simulink model "PIL_System_POTS"  (R2025b)
settings: Solver=FixedStepAuto  StartTime=0.0  StopTime=10.0  RelTol=1e-3  EnableMultiTasking=on
libraries: stm32f4xxblockslib x2
settings Model: STM32="{\"AnalogInput\":[{\"ID\":\"PIL_System_POTS:37\"},{\"ID\":\"PIL_System_POTS:38\"}]}"  Creator=Lakshay Taneja  LastModifiedBy=Lakshay Taneja
settings OptimizationCC: DefaultParameterBehavior=Inlined  EnhancedBackFolding=on  PassReuseOutputArgsAs=Individual arguments  ZeroExternalMemoryAtStartup=off  ZeroInternalMemoryAtStartup=off  MaxStackSize=512  OptimizeBlockOrder=speed  DifferentSizesBufferReuse=on  OptimizationCustomize=off  EfficientTunableParamExpr=on
settings DebuggingCC: ParameterTunabilityLossMsg=error
settings HardwareCC: ProdBitPerPointer=32.0  ProdBitPerSizeT=32.0  ProdBitPerPtrDiffT=32.0  ProdLargestAtomicInteger=Long  ProdLargestAtomicFloat=Double  ProdWordSize=32.0  ProdLongLongMode=on  ProdHWDeviceType=ARM Compatible->ARM Cortex-M
settings SFSimCC: MATLABDynamicMemAlloc=off
settings RTWCC: SystemTargetFile=ert.tlc  HardwareBoard=STM32F4xx Based  TemplateMakefile=ert_default_tmf  Toolchain=GNU Tools for ARM Embedded Processors  CreateSILPILBlock=PIL  Description=Embedded Coder
settings CodeAppCC: ForceParamTrailComments=on  IgnoreCustomStorageClasses=off  OperatorAnnotations=on  SimulinkDataObjDesc=on  SFDataObjDesc=on  InsertBlockDesc=on
settings ERTTargetCC: ExtModeTransport=3.0  ExtModeStaticAlloc=on  ExtModeStaticAllocSize=2048.0  ExtModeMexFile=ext_xcp  ExtModeIntrfLevel=Level2 - Open  TargetLangStandard=C99 (ISO)  CodeReplacementLibrary=ARM Cortex-M

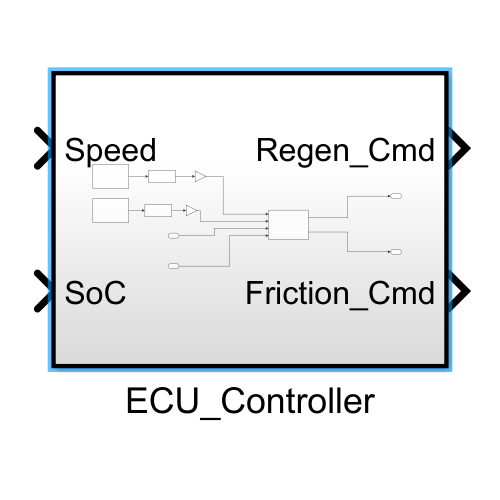
[thumbnail: Simulink's stored preview of the top-level diagram]
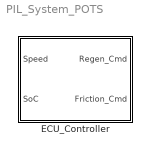
== system PIL_System_POTS ==
  ECU_Controller : Subsystem  TreatAsAtomicUnit=on

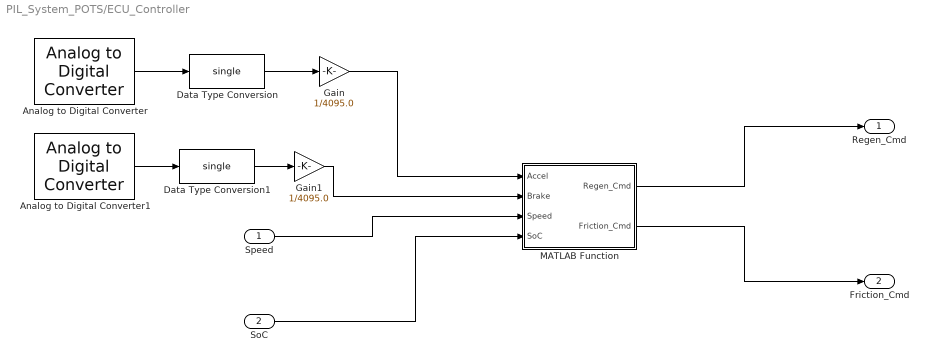
== system PIL_System_POTS/ECU_Controller ==
  Speed : Inport  OutDataTypeStr=single
  SoC : Inport  Port=2  OutDataTypeStr=single
  Analog to Digital Converter : stm32f4xxblockslib/Analog to Digital Converter  ADCModule=ADC1  ConversionGroup=Regular  TriggerMode=Trigger and read  NumberOfConversions=1  EnableBufferConv=off  BufferLength=1  OutputStatus=off  SampleTime=0.01  EnableSimPort=off  hoistedMaskSrc=ECSoC/ECSimCodegen/Analog to Digital Converter
      settings: LibrarySourceBlock=stm32f1xxblockslib/Analog to Digital Converter
  Analog to Digital Converter1 : stm32f4xxblockslib/Analog to Digital Converter  ADCModule=ADC2  ConversionGroup=Regular  TriggerMode=Trigger and read  NumberOfConversions=1  EnableBufferConv=off  BufferLength=1  OutputStatus=off  SampleTime=0.01  EnableSimPort=off  hoistedMaskSrc=ECSoC/ECSimCodegen/Analog to Digital Converter
      settings: LibrarySourceBlock=stm32f1xxblockslib/Analog to Digital Converter
  Data Type Conversion : DataTypeConversion  OutDataTypeStr=single  SaturateOnIntegerOverflow=off  RndMeth=Floor
  Data Type Conversion1 : DataTypeConversion  OutDataTypeStr=single  SaturateOnIntegerOverflow=off  RndMeth=Floor
  Gain : Gain  Gain=1/4095.0  OutDataTypeStr=single
  Gain1 : Gain  Gain=1/4095.0  OutDataTypeStr=single
  MATLAB Function : MATLAB Function  TreatAsAtomicUnit=on
  Regen_Cmd : Outport  OutDataTypeStr=single
  Friction_Cmd : Outport  Port=2  OutDataTypeStr=single
  wires:
  Speed/1 -> MATLAB Function/3(Speed)
  MATLAB Function/2(Friction_Cmd) -> Friction_Cmd/1
  MATLAB Function/1(Regen_Cmd) -> Regen_Cmd/1
  SoC/1 -> MATLAB Function/4(SoC)
  Analog to Digital Converter/1 -> Data Type Conversion/1
  Analog to Digital Converter1/1 -> Data Type Conversion1/1
  Gain/1 -> MATLAB Function/1(Accel)
  Gain1/1 -> MATLAB Function/2(Brake)
  Data Type Conversion/1 -> Gain/1
  Data Type Conversion1/1 -> Gain1/1

== matlab function PIL_System_POTS/ECU_Controller/MATLAB Function ==
  data: Accel input; Regen_Cmd output; Brake input; Speed input; SoC input; Friction_Cmd output
function [Regen_Cmd, Friction_Cmd] = ECU_Logic(Accel, Brake, Speed, SoC)
    % --- 0. SAFETY INITIALIZATION ---
    Regen_Cmd    = single(0);
    Friction_Cmd = single(0);

    % --- 1. FORCE INPUTS TO SINGLE ---
    ac_in = single(Accel);
    br_in = single(Brake);
    sp_in = single(Speed);
    sc_in = single(SoC);

    % --- 2. "SPORT HYBRID" PARAMETERS ---
    
    % Propulsion: 2800 Nm (Strong acceleration)
    Max_Prop_Trq    = single(2800);  
    
    % Braking: -4500 Nm (Emergency stopping power)
    Max_Brake_Trq   = single(-4500); 
    
    % One-Pedal: -300 Nm (THE SWEET SPOT)
    % Strong enough to charge battery, but smooth enough to glide.
    One_Pedal_Trq   = single(-300);       
    
    % Deadband: 0.05 (CRITICAL FIX)
    % Ignores the first 5% of knob rotation to prevent "Ghost Braking"
    Deadband        = single(0.05);
    
    Zero            = single(0);
    Soc_Max         = single(0.95);
    
    % Speed Governor: 45 m/s (~162 km/h)
    Top_Speed_Limit = single(45.0); 

    % --- 3. LOGIC VARIABLES ---
    req_prop    = single(0);
    req_oneped  = single(0);
    req_brake   = single(0);
    calc_regen  = single(0);
    calc_frict  = single(0);
    
    % --- 4. DRIVER INTENT ---
    
    % A. Propulsion
    if ac_in > Deadband
        if sp_in < Top_Speed_Limit
            req_prop = ac_in * Max_Prop_Trq;
            % Soft Limiter (Fade out torque 5 m/s before top speed)
            if sp_in > (Top_Speed_Limit - single(5.0))
                factor = (Top_Speed_Limit - sp_in) / single(5.0);
                req_prop = req_prop * factor;
            end
        else
            req_prop = Zero;
        end
        is_coasting = false; 
    else
        req_prop = Zero;
        is_coasting = true;
    end
    
    % B. One-Pedal Logic (Active when coasting)
    if is_coasting
        req_oneped = One_Pedal_Trq;
    else
        req_oneped = Zero;
    end
    
    % C. Friction Brake Request
    if br_in > Deadband
        req_brake = br_in * Max_Brake_Trq;
    else
        req_brake = Zero;
    end
    
    % D. Total Request
    total_req = single(req_prop + req_oneped + req_brake);
    
    
    % --- 5. SYSTEM CONSTRAINTS ---
    x_spd = single([0,    5,     10,    25,    45]); 
    y_trq = single([0, -1000, -2500, -2500, -1200]); 
    
    max_regen_lim = single(interp1(x_spd, y_trq, sp_in, 'linear', 'extrap'));
    
    if sc_in > Soc_Max
        avail_regen = Zero;
    else
        avail_regen = max_regen_lim;
    end
    
    
    % --- 6. TORQUE SPLIT ---
    if total_req >= Zero
        calc_regen = total_req;
        calc_frict = Zero;
    else
        % BRAKING
        calc_regen = max(total_req, avail_regen);
        calc_frict = total_req - calc_regen;
    end
    
    % --- 7. OUTPUTS ---
    Regen_Cmd    = single(calc_regen);
    Friction_Cmd = single(calc_frict);
end
